simulink model "exertConstForce"  (Simulink 7.5)
settings: Solver=ode1  StartTime=0.0  StopTime=Inf  FixedStep=0.001  RelTol=1e-3
PostLoadFcn:
  | , if any(exist('dsrtsu_mdlpostloadfcn', 'file') == [2, 3, 6]), try dsrtsu_mdlpostloadfcn('Execute', bdroot); catch fprintf('Error in PostLoadFcn (dsrtsu_mdlpostloadfcn) for model "%s":\n %s\n', bdroot, lasterr); end, end,
values from neighbouring files (symbols this model uses):
  calMatrix = csvread('calibration.csv')    [main.m]
libraries: rtilib1103 x9, dspindex x1, simulink x1
settings Model: DSRTSU_INTERNAL_RTI_VER=360  DSRTSU_INTERNAL_RTI_TYPE=rti1103  Creator=daq  LastModifiedBy=daq  BufferReuse=off
settings OptimizationCC: BlockReduction=off  OptimizeBlockIOStorage=off  BufferReuse=off  ExpressionFolding=off  LocalBlockOutputs=off
settings HardwareCC: ProdIntDivRoundTo=Zero  ProdEndianess=BigEndian  ProdHWDeviceType=Generic->Custom  TargetIntDivRoundTo=Zero  TargetEndianess=BigEndian  TargetHWDeviceType=Generic->Custom
settings RTWCC: SystemTargetFile=rti1103.tlc  MakeCommand=make_rti  TemplateMakefile=rti1103.tmf  Description=dSPACE DS1103 Hardware Platform  ProcessScript=rti1103_make_rtw_hook
settings STFCustomTargetCC: ParMdlRefBuildCompliant=on  GeneratePreprocessorConditionals=Disable all  SystemTargetFile=rti1103.tlc
settings GRTTargetCC: CompOptLevelCompliant=off  MatFileLogging=off  ExtModeMexFile=noextcomm
settings CustomProperty: DataType=RTWOptions_EnumType_C__dSPACE_matlab_rti1103_tlc_rti1103_1InitialSimState  Value=RUN
settings EnumStrPairs: String=RUN

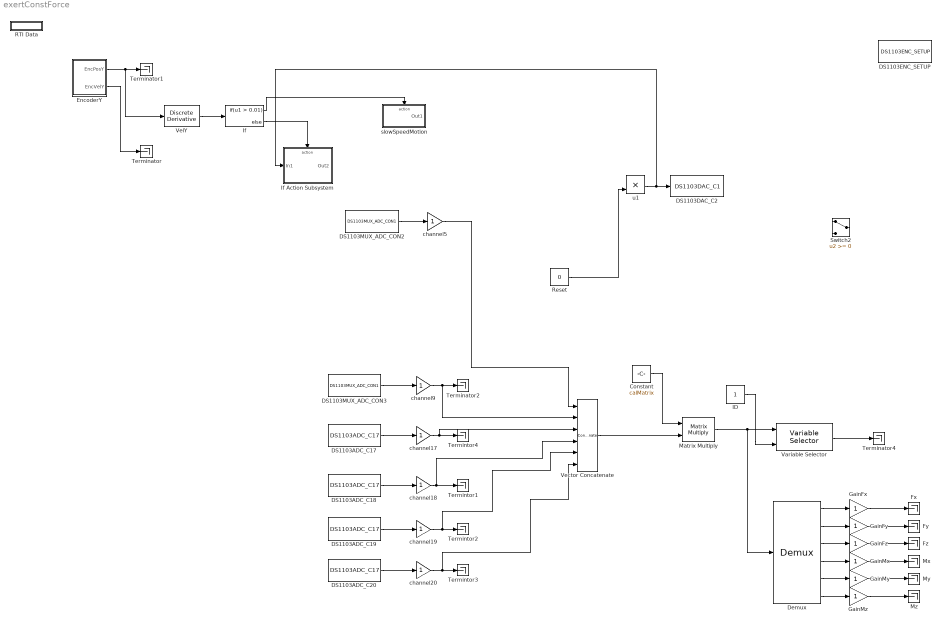
== system exertConstForce ==
  Constant : Constant  Value=calMatrix  OutDataType=fixdt(1, 16)  OutScaling=2^0
  DS1103ADC_C17 : rtilib1103/DS1103 MASTER PPC/DS1103ADC_C17  SystemSampleTime=-1  ChannelNo=17  TimerAPreTrigger=0  Reserved2=[]  Reserved3=[]  Reserved4=[]  DialogFcn=gui1103adc  UnitName={ 'DS1103ADC_C' }  UnitValues={ 17 }  DSProperties=struct('RTI',struct('Version',uint32(1),'BlockType',struct('isSLSource',uint8(1),'isSLSink',uint8(0),'isHWSource',uint8(1),'isHWSink',uint8(0),'isSetup',uint8(0),'isInline',uint8(1),'isNonInline',uint8(0),'isInterrupt',uint8(0),'isChannelwise',uint8(1)),'IOBoardType','DS1103MASTER','UnitType','ADC','Identifier','ADC','DialogType','ML','BlockSet','NONE','SlaveProcessor','NONE'))
  DS1103ADC_C18 : rtilib1103/DS1103 MASTER PPC/DS1103ADC_C17  SystemSampleTime=-1  ChannelNo=18  TimerAPreTrigger=0  Reserved2=[]  Reserved3=[]  Reserved4=[]  DialogFcn=gui1103adc  UnitName={ 'DS1103ADC_C' }  UnitValues={ 18 }  DSProperties=struct('RTI',struct('Version',uint32(1),'BlockType',struct('isSLSource',uint8(1),'isSLSink',uint8(0),'isHWSource',uint8(1),'isHWSink',uint8(0),'isSetup',uint8(0),'isInline',uint8(1),'isNonInline',uint8(0),'isInterrupt',uint8(0),'isChannelwise',uint8(1)),'IOBoardType','DS1103MASTER','UnitType','ADC','Identifier','ADC','DialogType','ML','BlockSet','NONE','SlaveProcessor','NONE'))
  DS1103ADC_C19 : rtilib1103/DS1103 MASTER PPC/DS1103ADC_C17  SystemSampleTime=-1  ChannelNo=19  TimerAPreTrigger=0  Reserved2=[]  Reserved3=[]  Reserved4=[]  DialogFcn=gui1103adc  UnitName={ 'DS1103ADC_C' }  UnitValues={ 19 }  DSProperties=struct('RTI',struct('Version',uint32(1),'BlockType',struct('isSLSource',uint8(1),'isSLSink',uint8(0),'isHWSource',uint8(1),'isHWSink',uint8(0),'isSetup',uint8(0),'isInline',uint8(1),'isNonInline',uint8(0),'isInterrupt',uint8(0),'isChannelwise',uint8(1)),'IOBoardType','DS1103MASTER','UnitType','ADC','Identifier','ADC','DialogType','ML','BlockSet','NONE','SlaveProcessor','NONE'))
  DS1103ADC_C20 : rtilib1103/DS1103 MASTER PPC/DS1103ADC_C17  SystemSampleTime=-1  ChannelNo=20  TimerAPreTrigger=0  Reserved2=[]  Reserved3=[]  Reserved4=[]  DialogFcn=gui1103adc  UnitName={ 'DS1103ADC_C' }  UnitValues={ 20 }  DSProperties=struct('RTI',struct('Version',uint32(1),'BlockType',struct('isSLSource',uint8(1),'isSLSink',uint8(0),'isHWSource',uint8(1),'isHWSink',uint8(0),'isSetup',uint8(0),'isInline',uint8(1),'isNonInline',uint8(0),'isInterrupt',uint8(0),'isChannelwise',uint8(1)),'IOBoardType','DS1103MASTER','UnitType','ADC','Identifier','ADC','DialogType','ML','BlockSet','NONE','SlaveProcessor','NONE'))
  DS1103DAC_C2 : rtilib1103/DS1103 MASTER PPC/DS1103DAC_C1  SystemSampleTime=-1  ChannelNo=2  InitValue=0  TermMode=1  TermValue=0  Reserved1=[]  Reserved2=[]  Reserved3=[]  Reserved4=[]  DialogFcn=gui1103dac  UnitName={ 'DS1103DAC_C' }  UnitValues={ 2 }  DSProperties=struct('RTI',struct('Version',uint32(1),'BlockType',struct('isSLSource',uint8(0),'isSLSink',uint8(1),'isHWSource',uint8(0),'isHWSink',uint8(1),'isSetup',uint8(0),'isInline',uint8(1),'isNonInline',uint8(0),'isInterrupt',uint8(0),'isChannelwise',uint8(1)),'IOBoardType','DS1103MASTER','UnitType','DAC','Identifier','DAC','DialogType','ML','BlockSet','NONE','SlaveProcessor','NONE'))
  DS1103ENC_SETUP : rtilib1103/DS1103 MASTER PPC/DS1103ENC_SETUP  SystemSampleTime=-1  EncRange=0  Reserved1=[]  Reserved2=[]  Reserved3=[]  Reserved4=[]  DialogFcn=gui1103enc_setup  UnitName={ 'DS1103ENC_SETUP' }  UnitValues={ [] }  DSProperties=struct('RTI',struct('Version',uint32(1),'BlockType',struct('isSLSource',uint8(0),'isSLSink',uint8(0),'isHWSource',uint8(0),'isHWSink',uint8(0),'isSetup',uint8(0),'isInline',uint8(1),'isNonInline',uint8(0),'isInterrupt',uint8(0),'isChannelwise',uint8(0)),'IOBoardType','DS1103MASTER','UnitType','ENC','Identifier','ENCMASTER','DialogType','ML','BlockSet','NONE','SlaveProcessor','NONE'))
      settings: SignalType=[0 0 0 0 0 0 0]
  DS1103MUX_ADC_CON2 : rtilib1103/DS1103 MASTER PPC/DS1103MUX_ADC_CON1  SystemSampleTime=-1  ConverterNo=2  ChannelNos=1  TimerAPreTrigger=0  Reserved2=[]  Reserved3=[]  Reserved4=[]  DialogFcn=gui1103mux_adc  UnitName={ 'DS1103MUX_ADC_CON' }  UnitValues={ 2 }  DSProperties=struct('RTI',struct('Version',uint32(1),'BlockType',struct('isSLSource',uint8(1),'isSLSink',uint8(0),'isHWSource',uint8(1),'isHWSink',uint8(0),'isSetup',uint8(0),'isInline',uint8(1),'isNonInline',uint8(0),'isInterrupt',uint8(0),'isChannelwise',uint8(0)),'IOBoardType','DS1103MASTER','UnitType','ADC','Identifier','ADCMUX','DialogType','ML','BlockSet','NONE','SlaveProcessor','NONE'))
  DS1103MUX_ADC_CON3 : rtilib1103/DS1103 MASTER PPC/DS1103MUX_ADC_CON1  SystemSampleTime=-1  ConverterNo=3  ChannelNos=1  TimerAPreTrigger=0  Reserved2=[]  Reserved3=[]  Reserved4=[]  DialogFcn=gui1103mux_adc  UnitName={ 'DS1103MUX_ADC_CON' }  UnitValues={ 3 }  DSProperties=struct('RTI',struct('Version',uint32(1),'BlockType',struct('isSLSource',uint8(1),'isSLSink',uint8(0),'isHWSource',uint8(1),'isHWSink',uint8(0),'isSetup',uint8(0),'isInline',uint8(1),'isNonInline',uint8(0),'isInterrupt',uint8(0),'isChannelwise',uint8(0)),'IOBoardType','DS1103MASTER','UnitType','ADC','Identifier','ADCMUX','DialogType','ML','BlockSet','NONE','SlaveProcessor','NONE'))
  Demux : Demux  Outputs=6
  EncoderY : Subsystem
  Fx : Terminator
  Fy : Terminator
  Fz : Terminator
  GainFx : Gain  ParameterDataType=fixdt(1, 16)  ParameterScaling=2^0  OutDataType=fixdt(1, 16)  OutScaling=2^0
  GainFy : Gain  ParameterDataType=fixdt(1, 16)  ParameterScaling=2^0  OutDataType=fixdt(1, 16)  OutScaling=2^0
  GainFz : Gain  ParameterDataType=fixdt(1, 16)  ParameterScaling=2^0  OutDataType=fixdt(1, 16)  OutScaling=2^0
  GainMx : Gain  ParameterDataType=fixdt(1, 16)  ParameterScaling=2^0  OutDataType=fixdt(1, 16)  OutScaling=2^0
  GainMy : Gain  ParameterDataType=fixdt(1, 16)  ParameterScaling=2^0  OutDataType=fixdt(1, 16)  OutScaling=2^0
  GainMz : Gain  ParameterDataType=fixdt(1, 16)  ParameterScaling=2^0  OutDataType=fixdt(1, 16)  OutScaling=2^0
  ID : Constant  OutDataType=fixdt(1, 16)  OutScaling=2^0
  If : If  IfExpression=u1 > 0.01
  If Action Subsystem : Subsystem  TreatAsAtomicUnit=on
  Matrix Multiply : Product  Multiplication=Matrix(*)  OutDataType=sfix(16)  OutScaling=2^0
  Mx : Terminator
  My : Terminator
  Mz : Terminator
  RTI Data : Subsystem  Tag=struct('RTIDataServer',struct('RTIDataServerVs','2','RTIModelDescription','struct(''main'',''exertConstForce'',''sub'','''',''isMp'',0)'))  LoadFcn="if exist('rtidc'), try,  rtidc('DataHostBlockClbLoad', gcbh); catch, disp(['Warning: ''LoadFcn'' for RTI Data block failed: ' lasterr]); end, end,"
      settings: CopyFcn="if exist('rtidc'), try,  rtidc('DataHostBlockClbCopy', gcbh); catch, disp(['Warning: ''CopyFcn'' for RTI Data block failed: ' lasterr]); end, end,"  DeleteFcn="if exist('rtidc'), try,  rtidc('DataHostBlockClbDelete', gcbh); catch, disp(['Warning: ''DeleteFcn'' for RTI Data block failed: ' lasterr]); end, end,"  ModelCloseFcn="if exist('rtidc'), try,  rtidc('DataHostBlockClbModelClose', gcbh); catch, disp(['Warning: ''ModelCloseFcn'' for RTI Data block failed: ' lasterr]); end, end,"  PreSaveFcn="if exist('rtidc'), try,  rtidc('DataHostBlockClbPreSave', gcbh); catch, disp(['Warning: ''PreSaveFcn'' for RTI Data block failed: ' lasterr]); end, end,"  PostSaveFcn="if exist('rtidc'), try,  rtidc('DataHostBlockClbPostSave', gcbh); catch, disp(['Warning: ''PostSaveFcn'' for RTI Data block failed: ' lasterr]); end, end,"  NameChangeFcn="if exist('rtidc'), try,  rtidc('DataHostBlockClbNameChange', gcbh); catch, disp(['Warning: ''NameChangeFcn'' for RTI Data block failed: ' lasterr]); end, end,"
      mask Type: RTI_DATA_HOST
      mask Description:
      | RTI Data Block.
      | This block is used by RTI to store internal model-dependent data.
      | Please keep this block on the root level of the model. Deleting this block will result in data loss.
      | 
      | NEVER DELETE OR COPY THIS BLOCK!
      mask Help:
      | RTI Data Block.
      | This block is used by RTI to store internal model-dependent data.
      | Please keep this block on the root level of the model. Deleting this block will result in data loss.
      | 
      | NEVER DELETE OR COPY THIS BLOCK!
      mask Display:
      | text(0.5, 0.5, 'RTI Data', 'HorizontalAlignment', 'center');
      | plot([1 0]);
  Reset : Constant  Value=0  OutDataType=fixdt(1, 16)  OutScaling=2^0
  Switch2 : Switch  OutDataType=fixdt(1, 16)  OutScaling=2^0
  Terminator{,1..2,4} (4 alike) : Terminator
  Termintor{1..4} (4 alike) : Terminator
  Variable Selector : dspindex/Variable Selector  NumInputs=1  rowsOrCols=Rows  IdxMode=Variable  Elements=[1 3]  ZerOneIdxMode=One-based  errmode=Clip Index  FillMode=on  FillValues=0
  Vector Concatenate : Concatenate  NumInputs=6  Mode=Vector
  VelY : simulink/Discrete/Discrete Derivative  SystemSampleTime=-1  gainval=1.0  ICPrevScaledInput=0.0  OutMin=[]  OutMax=[]  OutDataType=fixdt(1, 16)  OutScaling=2^-10  DoSatur=off
  channel{5,9,17..20} (6 alike) : Gain  ParameterDataType=fixdt(1, 16)  ParameterScaling=2^0  OutDataType=fixdt(1, 16)  OutScaling=2^0
  slowSpeedMotion : Subsystem  TreatAsAtomicUnit=on
  u1 : Product  OutDataType=fixdt(1, 16)  OutScaling=2^0  RndMeth=Zero
  wires:
  EncoderY/1(EncPosY) -> Terminator1/1, VelY/1
  EncoderY/2(EncVelY) -> Terminator/1
  VelY/1 -> If/1
  DS1103MUX_ADC_CON2/1 -> channel5/1
  channel5/1 -> Vector Concatenate/1
  Reset/1 -> u1/2
  u1/1 -> DS1103DAC_C2/1, If Action Subsystem/1(In1)
  DS1103MUX_ADC_CON3/1 -> channel9/1
  channel9/1 -> Terminator2/1, Vector Concatenate/2
  channel17/1 -> Termintor4/1, Vector Concatenate/3
  DS1103ADC_C17/1 -> channel17/1
  channel18/1 -> Termintor1/1, Vector Concatenate/4
  DS1103ADC_C18/1 -> channel18/1
  channel19/1 -> Termintor2/1, Vector Concatenate/5
  DS1103ADC_C19/1 -> channel19/1
  channel20/1 -> Termintor3/1, Vector Concatenate/6
  DS1103ADC_C20/1 -> channel20/1
  Constant/1 -> Matrix Multiply/1
  Vector Concatenate/1 -> Matrix Multiply/2
  Matrix Multiply/1 -> Variable Selector/1, Demux/1
  ID/1 -> Variable Selector/2
  Variable Selector/1 -> Terminator4/1
  Demux/1 -> GainFx/1
  Demux/2 -> GainFy/1
  Demux/3 -> GainFz/1
  Demux/4 -> GainMx/1
  Demux/5 -> GainMy/1
  Demux/6 -> GainMz/1
  GainFx/1 -> Fx/1
  GainFy/1 -> Fy/1
  GainFz/1 -> Fz/1
  GainMx/1 -> Mx/1
  GainMy/1 -> My/1
  GainMz/1 -> Mz/1
  If/1 -> slowSpeedMotion/Action
  If/2 -> If Action Subsystem/Action

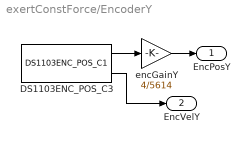
== system exertConstForce/EncoderY ==
  DS1103ENC_POS_C3 : rtilib1103/DS1103 MASTER PPC/DS1103ENC_POS_C1  SystemSampleTime=-1  ChannelNo=3  PosValue=0  Reserved1=[]  Reserved2=[]  Reserved3=[]  Reserved4=[]  DialogFcn=gui1103enc_pos  UnitName={ 'DS1103ENC_POS_C' }  UnitValues={3}  DSProperties=struct('RTI',struct('Version',uint32(1),'BlockType',struct('isSLSource',uint8(1),'isSLSink',uint8(0),'isHWSource',uint8(1),'isHWSink',uint8(0),'isSetup',uint8(0),'isInline',uint8(1),'isNonInline',uint8(0),'isInterrupt',uint8(0),'isChannelwise',uint8(1)),'IOBoardType','DS1103MASTER','UnitType','ENC','Identifier','ENCPOSCH','DialogType','ML','BlockSet','NONE','SlaveProcessor','NONE'))
  encGainY : Gain  Gain=4/5614  ParameterDataType=fixdt(1, 16)  ParameterScaling=2^0  OutDataType=fixdt(1, 16)  OutScaling=2^0
  EncPosY : Outport
  EncVelY : Outport  Port=2  OutDataType=fixdt(1, 16)  OutScaling=2^0
  wires:
  DS1103ENC_POS_C3/1 -> encGainY/1
  encGainY/1 -> EncPosY/1
  DS1103ENC_POS_C3/2 -> EncVelY/1

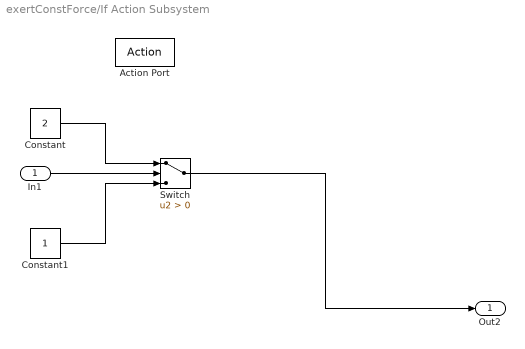
== system exertConstForce/If Action Subsystem ==
  In1 : Inport  OutDataType=fixdt(1, 16)  OutScaling=2^0
  Action Port : ActionPort  ActionType=else
  Constant : Constant  Value=2  OutDataType=fixdt(1, 16)  OutScaling=2^0
  Constant1 : Constant  OutDataType=fixdt(1, 16)  OutScaling=2^0
  Switch : Switch  Criteria=u2 > Threshold  OutDataType=fixdt(1, 16)  OutScaling=2^0
  Out2 : Outport  OutDataType=fixdt(1, 16)  OutScaling=2^0
  wires:
  In1/1 -> Switch/2
  Constant/1 -> Switch/1
  Constant1/1 -> Switch/3
  Switch/1 -> Out2/1

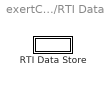
== system exertConstForce/RTI Data ==
  RTI Data Store : Subsystem  Tag="struct('private',struct('version',struct('dsVer',uint32(2),'dsVerCreation',uint32(2),'RTI',struct('ver','6.5','type','RTI1103')),'access',struct('type','Model','isPerm',1,'created',['13-Sep-2016 15:06:26'],'modified',['07-Oct-2016 16:36:46'],'location','')),'public',struct('main',struct('data',[]),'sub',struct('name',{{'exertConstForce'}},'data',{{struct('TH',struct('thTaskInfo',struct('taskType',{'TIMER','HWINT','TMRINT','SWINT'},'tasksNumOf',{1,0,0,0},'srcIds',{{'TIMERA'},{},{},{}},'taskNames',{{['Timer Task 1']},{},{},{}})),'th_tc',struct('dataType','TASK','taskGroupId','','taskGroupList',{{}},'taskSchedulingPolicy','FCFS','taskType','TIMER','blkh',-1,'srcId','TIMERA','srcSgnName',['Timer A interrupt'],'srcCpuName','','taskName',['Timer Task 1  [0.001] s'],'taskNameDisplayExt','','smplTime',0.001,'smplTimeOffs',0,'hasFixedPriority',0,'priority',1,'hasFixedOvc',0,'ovcType',1,'ovcMax',1),'tc_th',struct('dataType','TASK','taskGroupId','','taskGroupList',{{}},'taskSchedulingPolicy','FCFS','taskType','TIMER','blkh',-1,'srcId','TIMERA','srcSgnName',['Timer A interrupt'],'srcCpuName','','taskName',['Timer Task 1  [0.001] s'],'taskNameDisplayExt','','smplTime',0.001,'smplTimeOffs',0,'hasFixedPriority',0,'priority',1,'hasFixedOvc',0,'ovcType',1,'ovcMax',1))}})))"
      mask Type: RTI_DATA_STORE
      mask Description:
      | RTI Data Store Block. This block is used by RTI to store internal model dependent data. Deleting this block will result in data loss.
      | 
      | NEVER DELETE, COPY, OR MODIFY THIS BLOCK!
      mask Help:
      | RTI Data Store Block. This block is used by RTI to store internal model dependent data. Deleting this block will result in data loss.
      | 
      | NEVER DELETE, COPY, OR MODIFY THIS BLOCK!
      mask Display: text(0.5, 0.5, ' ', 'HorizontalAlignment', 'center');

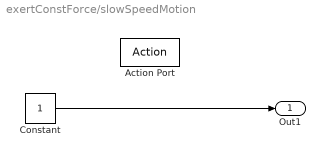
== system exertConstForce/slowSpeedMotion ==
  Action Port : ActionPort  ActionType=then
  Constant : Constant  OutDataType=fixdt(1, 16)  OutScaling=2^0
  Out1 : Outport  OutDataType=fixdt(1, 16)  OutScaling=2^0
  wires:
  Constant/1 -> Out1/1

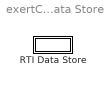
== system exertConstForce/RTI Data/RTI Data Store ==
  RTI Data Store : Subsystem
      mask Type: RTI_DATA_STORE
      mask Description:
      | RTI Data Store Block. This block is used by RTI to store internal model dependent data. Deleting this block will result in data loss.
      | 
      | NEVER DELETE, COPY, OR MODIFY THIS BLOCK!
      mask Help:
      | RTI Data Store Block. This block is used by RTI to store internal model dependent data. Deleting this block will result in data loss.
      | 
      | NEVER DELETE, COPY, OR MODIFY THIS BLOCK!
      mask Display: text(0.5, 0.5, ' ', 'HorizontalAlignment', 'center');

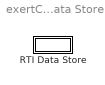
== system exertConstForce/RTI Data/RTI Data Store/RTI Data Store ==
  RTI Data Store : Subsystem
      mask Type: RTI_DATA_STORE
      mask Description:
      | RTI Data Store Block. This block is used by RTI to store internal model dependent data. Deleting this block will result in data loss.
      | 
      | NEVER DELETE, COPY, OR MODIFY THIS BLOCK!
      mask Help:
      | RTI Data Store Block. This block is used by RTI to store internal model dependent data. Deleting this block will result in data loss.
      | 
      | NEVER DELETE, COPY, OR MODIFY THIS BLOCK!
      mask Display: text(0.5, 0.5, ' ', 'HorizontalAlignment', 'center');

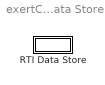
== system exertConstForce/RTI Data/RTI Data Store/RTI Data Store/RTI Data Store ==
  RTI Data Store : Subsystem
      mask Type: RTI_DATA_STORE
      mask Description:
      | RTI Data Store Block. This block is used by RTI to store internal model dependent data. Deleting this block will result in data loss.
      | 
      | NEVER DELETE, COPY, OR MODIFY THIS BLOCK!
      mask Help:
      | RTI Data Store Block. This block is used by RTI to store internal model dependent data. Deleting this block will result in data loss.
      | 
      | NEVER DELETE, COPY, OR MODIFY THIS BLOCK!
      mask Display: text(0.5, 0.5, ' ', 'HorizontalAlignment', 'center');

== system exertConstForce/RTI Data/RTI Data Store/RTI Data Store/RTI Data Store/RTI Data Store ==
